simulink model "current"  (R2023b)
settings: Solver=VariableStepAuto  StartTime=0.0  StopTime=0.02  RelTol=1e-3
settings Model: Creator=George  LastModifiedBy=volko

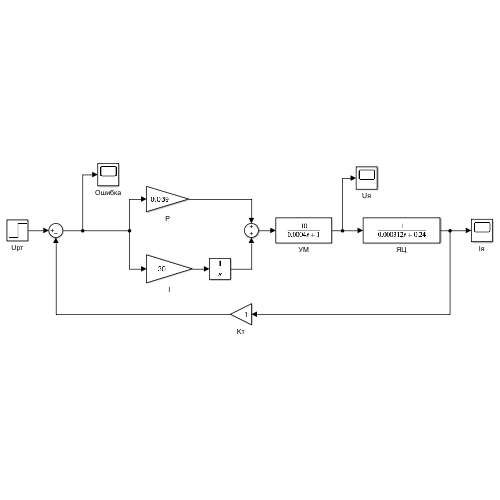
[thumbnail: Simulink's stored preview of the top-level diagram]
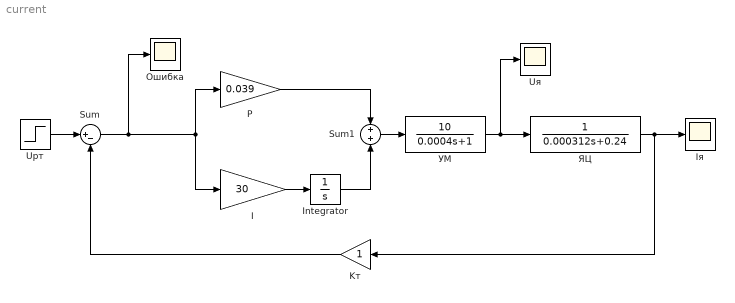
== system current ==
  I : Gain  Gain=30
  Integrator : Integrator
  Iя : Scope
  Kт : Gain
  P : Gain  Gain=0.039
  Sum : Sum  Inputs=|+-
  Sum1 : Sum
  Uрт : Step  Time=0  SampleTime=0
  Uя : Scope
  Ошибка : Scope
  УМ : TransferFcn  Numerator=[10]  Denominator=[0.0004 1]
  ЯЦ : TransferFcn  Denominator=[0.000312 0.24]
  wires:
  Uрт/1 -> Sum/1
  I/1 -> Integrator/1
  Sum/1 -> Ошибка/1, I/1, P/1
  P/1 -> Sum1/1
  Integrator/1 -> Sum1/2
  Sum1/1 -> УМ/1
  УМ/1 -> Uя/1, ЯЦ/1
  ЯЦ/1 -> Iя/1, Kт/1
  Kт/1 -> Sum/2
